simulink subsystem "KinematicSteering"  (R2023b)
settings: Solver=VariableStepAuto  StartTime=0.0  StopTime=10.0  RelTol=1e-3
undefined symbols (not defined in the file): PlntSteerRatio, PlntVehDstCGFrntAxl, PlntVehDstCGRearAxl, PlntVehTrckWdth
libraries: vehdynlibsteering x2
settings Model: ModifiedByFormat=The MathWorks, Inc.  Creator=The MathWorks, Inc.  LastModifiedBy=The MathWorks, Inc.

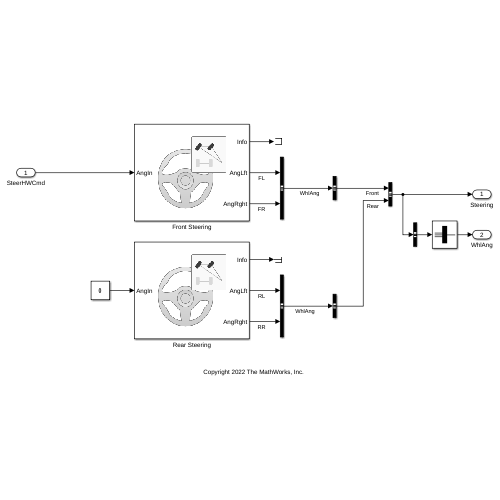
[thumbnail: Simulink's stored preview of the top-level diagram]
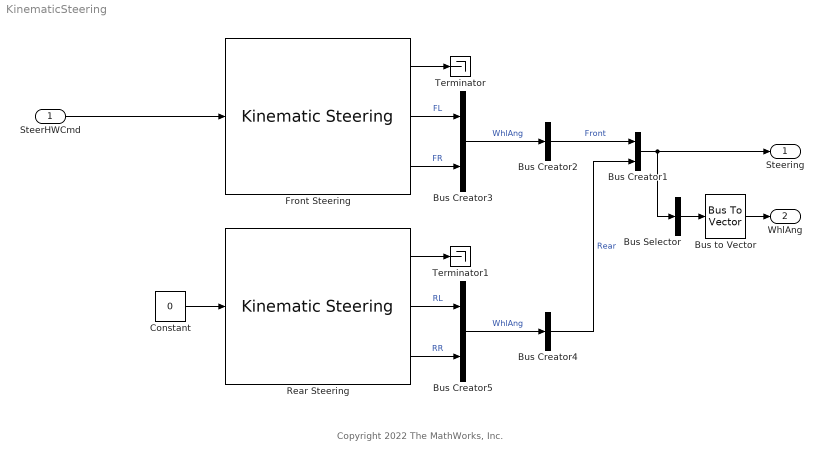
== system KinematicSteering ==
  note: Copyright 2022 The MathWorks, Inc.
  SteerHWCmd : Inport
  Bus Creator1 : BusCreator  Inputs=2
  Bus Creator2 : BusCreator  Inputs=1
  Bus Creator3 : BusCreator  Inputs=2
  Bus Creator4 : BusCreator  Inputs=1
  Bus Creator5 : BusCreator  Inputs=2
  Bus Selector : BusSelector  OutputSignals=Front.WhlAng.FL,Front.WhlAng.FR,Rear.WhlAng.RL,Rear.WhlAng.RR  OutputAsBus=on
  Bus to Vector : BusToVector
  Constant : Constant  Value=0  SampleTime=-1
  Front Steering : vehdynlibsteering/Kinematic Steering  StrgType=Ackerman  StrgRatioType=Constant  Loc=Front  NrmlFctr=1  TrckWdth=PlntVehTrckWdth(1)  WhlBase=PlntVehDstCGFrntAxl+PlntVehDstCGRearAxl  Db=0  StrgRng=PlntSteerRange  StrgAngBpts="[-6.2832   -5.0265   -3.7699   -2.5133   -1.2566         0    1.2566    2.5133    3.7699    5.0265    6.2832]"  StrgRatioTbl=|  StrgRatio=PlntSteerRatio  PctAckIn=off  PctAck=PlntSteerPctAck  PctAckTbl=ones(1,11)*100  StrgArmLngth=0.1  RckCsLngth=0.5  TieRodLngth=0.248128028933392  D=0.2  PnnRadius=0.0057  PnnRadiusTbl="[0.0055    0.0055    0.0056    0.0057    0.0057    0.0057    0.0057    0.0057    0.0056    0.0055    0.0055]"  RodLngth=0.1  ParaArmLngth=0.9  aMode=2
      | [13.5000   13.3750   13.2500   13.1250   13.0000   13.0000   13.0000   13.1250   13.2500   13.3750   13.5000
      | ]
  Rear Steering : vehdynlibsteering/Kinematic Steering  StrgType=Ackerman  StrgRatioType=Constant  Loc=Rear  NrmlFctr=1  TrckWdth=PlntVehTrckWdth(2)  WhlBase=PlntVehDstCGFrntAxl+PlntVehDstCGRearAxl  Db=0  StrgRng=10*pi/180  StrgAngBpts="[-6.2832   -5.0265   -3.7699   -2.5133   -1.2566         0    1.2566    2.5133    3.7699    5.0265    6.2832]"  StrgRatioTbl=|  StrgRatio=PlntSteerRatio*10  PctAckIn=off  PctAck=PlntSteerPctAck  PctAckTbl=ones(1,11)*100  StrgArmLngth=0.1  RckCsLngth=0.5  TieRodLngth=0.248128028933392  D=0.2  PnnRadius=0.0057  PnnRadiusTbl="[0.0055    0.0055    0.0056    0.0057    0.0057    0.0057    0.0057    0.0057    0.0056    0.0055    0.0055]"  RodLngth=0.1  ParaArmLngth=0.9  aMode=2
      | [13.5000   13.3750   13.2500   13.1250   13.0000   13.0000   13.0000   13.1250   13.2500   13.3750   13.5000
      | ]
  Terminator : Terminator
  Terminator1 : Terminator
  Steering : Outport  VectorParamsAs1DForOutWhenUnconnected=off
  WhlAng : Outport  Port=2  VectorParamsAs1DForOutWhenUnconnected=off
  wires:
  SteerHWCmd/1 -> Front Steering/1
  Front Steering/2 -> Bus Creator3/1  "FL"
  Front Steering/3 -> Bus Creator3/2  "FR"
  Constant/1 -> Rear Steering/1
  Bus Creator3/1 -> Bus Creator2/1  "WhlAng"
  Bus Creator1/1 -> Steering/1, Bus Selector/1
  Bus Creator2/1 -> Bus Creator1/1  "Front"
  Bus Creator4/1 -> Bus Creator1/2  "Rear"
  Bus Creator5/1 -> Bus Creator4/1  "WhlAng"
  Rear Steering/2 -> Bus Creator5/1  "RL"
  Rear Steering/3 -> Bus Creator5/2  "RR"
  Front Steering/1 -> Terminator/1
  Rear Steering/1 -> Terminator1/1
  Bus Selector/1 -> Bus to Vector/1
  Bus to Vector/1 -> WhlAng/1
